simulink model "aa_IOT"  (R2024b)
settings: Solver=VariableStepAuto  StartTime=0.0  StopTime=0.05  RelTol=1e-3
undefined symbols (not defined in the file): Acid, Ion, Lead, Lithium, sigbuilder_block
libraries: spsBreakerLib x120, spsBatteryLib x82, spsSeriesRLCBranchLib x74, spsIdealSwitchLib x37, spsVoltageMeasurementLib x29, slpidlib x17, spsMosfetLib x17, spsPWMGeneratorDCDCLib x11, spsDiodeLib x10, spsIGBTLib x4, spsCurrentMeasurementLib x4, spsThreePhaseSeriesRLCLoadLib x2
(part 5 of 6)

== system aa_IOT/Grid/Wall charger Connection Box/DC-DC converter with battery controller/Battery controller ==
  Add1 : Sum  Inputs=+-
  Add2 : Sum  Inputs=+-
  Add3 : Sum  Inputs=+-
  Constant1 : Constant  Value=48
  Constant2 : Constant  Value=25.98
  Constant4 : Constant
  Current controller : slpidlib/PID Controller  Controller=PI  Form=Parallel  TimeDomain=Discrete-time  UseExternalTs=off  SampleTime=500e-6  IntegratorMethod=Forward Euler  FilterMethod=Forward Euler  ControllerParametersSource=internal  P=0.005  I=10  UseKiTs=off  D=0  UseExternalDerivativeSource=off  N=100  UseFilter=on  TunerSelectOption=Transfer Function Based (PID Tuner App)  InitialConditionSource=internal  InitialConditionForIntegrator=0.54  InitialConditionForFilter=0  DifferentiatorICPrevScaledInput=0  ExternalReset=none  TrackingMode=off  Kt=1  LimitOutput=on  SatLimitsSource=internal  UpperSaturationLimit=0.95  LowerSaturationLimit=0  LinearizeAsGain=on  AntiWindupMode=none  Kb=1  LimitIntegrator=off  UpperIntegratorSaturationLimit=inf  LowerIntegratorSaturationLimit=-inf  POutMin=[]  POutMax=[]  IOutMin=[]  IOutMax=[]  DOutMin=[]  DOutMax=[]  NOutMin=[]  NOutMax=[]  SumOutMin=[]  SumOutMax=[]  SaturationOutMin=[]  SaturationOutMax=[]  PParamMin=[]  PParamMax=[]  IParamMin=[]  IParamMax=[]  DParamMin=[]  DParamMax=[]  NParamMin=[]  NParamMax=[]  KbParamMin=[]  KbParamMax=[]  KtParamMin=[]  KtParamMax=[]  KbOutMin=[]  KbOutMax=[]  KtOutMin=[]  KtOutMax=[]  IntegratorOutMin=[]  IntegratorOutMax=[]  FilterOutMin=[]  FilterOutMax=[]  SumI1OutMin=[]  SumI1OutMax=[]  SumI2OutMin=[]  SumI2OutMax=[]  SumI3OutMin=[]  SumI3OutMax=[]  SumI4OutMin=[]  SumI4OutMax=[]  SumDOutMin=[]  SumDOutMax=[]  DifferentiatorOutMin=[]  DifferentiatorOutMax=[]  FilterDiffOutCoefMin=[]  FilterDiffOutCoefMax=[]  ReciprocalOutMin=[]  ReciprocalOutMax=[]  SumDenOutMin=[]  SumDenOutMax=[]  SumNumOutMin=[]  SumNumOutMax=[]  DivideOutMin=[]  DivideOutMax=[]  UdiffTsProdOutMin=[]  UdiffTsProdOutMax=[]  NTsProdOutMin=[]  NTsProdOutMax=[]  UintegralTsProdOutMin=[]  UintegralTsProdOutMax=[]  UngainTsProdOutMin=[]  UngainTsProdOutMax=[]  ClampingZeroOutDataTypeStr=Inherit: Inherit via back propagation  ClampingZeroOutMin=[]  ClampingZeroOutMax=[]  FilterDenConstantOutDataTypeStr=Inherit: Inherit via back propagation  FilterDenConstantOutMin=[]  FilterDenConstantOutMax=[]  PCopyOutDataTypeStr=Inherit: Inherit via back propagation  PCopyOutMin=[]  PCopyOutMax=[]  NCopyOutDataTypeStr=Inherit: Inherit via back propagation  NCopyOutMin=[]  NCopyOutMax=[]  IntegratorContinuousStateAttributes=''  IntegratorStateMustResolveToSignalObject=off  IntegratorRTWStateStorageClass=Auto  FilterContinuousStateAttributes=''  FilterStateMustResolveToSignalObject=off  FilterRTWStateStorageClass=Auto  ParallelPVariant=InternalParameters  IdealPVariant=Disabled  IVariant=InternalParameters  DVariant=Disabled  IntegratorVariant=Discrete  SatVariant=Enabled  AWVariant=Passthrough  PCopyVariant=Disabled  TRVariant=Disabled  FdbkBlocksVariant=Forward  IdealPFdbkVariant=Disabled  SatFdbkVariant=Disabled  DerivativeFilterVariant=Disabled  NVariant=Disabled  NCopyVariant=Disabled_SignalSpec  FilterICVariant=Disabled  IntegratorICVariant=InternalICs  ExternalResetVariant=Disabled  TRSumVariant=Passthrough  SumFdbkVariant=Disabled  SumVariant=Sum_PI  TsampFilterVariant=InternalTs  TsampNgainVariant=Passthrough  TsampIntegralVariant=Disabled_SignalSpec  ExternalSaturationOutDataTypeStr=Inherit: Same as second input  DerivativeSourceVariant=Disabled  PreIntVariant=InternalPreInt
  Display2 : Display
  Display3 : Display
  Display4 : Display
  Gain1 : Gain  Gain=-1
  NOT1 : Logic  Operator=NOT  IconShape=distinctive  AllPortsSameDT=off  OutDataTypeStr=boolean
  NOT3 : Logic  Operator=NOT  IconShape=distinctive  AllPortsSameDT=off  OutDataTypeStr=boolean
  PWM Generator (DC-DC)1 : spsPWMGeneratorDCDCLib/PWM Generator (DC-DC)  Fsw=10e3  Ts=5e-6
  Switch1 : Switch  Criteria=u2 > Threshold  SaturateOnIntegerOverflow=off  InputSameDT=off
  discharge controlled : slpidlib/PID Controller  Controller=PI  Form=Parallel  TimeDomain=Discrete-time  UseExternalTs=off  SampleTime=500e-6  IntegratorMethod=Forward Euler  FilterMethod=Forward Euler  ControllerParametersSource=internal  P=0.25  I=50  UseKiTs=off  D=0  UseExternalDerivativeSource=off  N=100  UseFilter=on  TunerSelectOption=Transfer Function Based (PID Tuner App)  InitialConditionSource=internal  InitialConditionForIntegrator=0  InitialConditionForFilter=0  DifferentiatorICPrevScaledInput=0  ExternalReset=none  TrackingMode=off  Kt=1  LimitOutput=on  SatLimitsSource=internal  UpperSaturationLimit=22  LowerSaturationLimit=0  LinearizeAsGain=on  AntiWindupMode=none  Kb=1  LimitIntegrator=off  UpperIntegratorSaturationLimit=inf  LowerIntegratorSaturationLimit=-inf  POutMin=[]  POutMax=[]  IOutMin=[]  IOutMax=[]  DOutMin=[]  DOutMax=[]  NOutMin=[]  NOutMax=[]  SumOutMin=[]  SumOutMax=[]  SaturationOutMin=[]  SaturationOutMax=[]  PParamMin=[]  PParamMax=[]  IParamMin=[]  IParamMax=[]  DParamMin=[]  DParamMax=[]  NParamMin=[]  NParamMax=[]  KbParamMin=[]  KbParamMax=[]  KtParamMin=[]  KtParamMax=[]  KbOutMin=[]  KbOutMax=[]  KtOutMin=[]  KtOutMax=[]  IntegratorOutMin=[]  IntegratorOutMax=[]  FilterOutMin=[]  FilterOutMax=[]  SumI1OutMin=[]  SumI1OutMax=[]  SumI2OutMin=[]  SumI2OutMax=[]  SumI3OutMin=[]  SumI3OutMax=[]  SumI4OutMin=[]  SumI4OutMax=[]  SumDOutMin=[]  SumDOutMax=[]  DifferentiatorOutMin=[]  DifferentiatorOutMax=[]  FilterDiffOutCoefMin=[]  FilterDiffOutCoefMax=[]  ReciprocalOutMin=[]  ReciprocalOutMax=[]  SumDenOutMin=[]  SumDenOutMax=[]  SumNumOutMin=[]  SumNumOutMax=[]  DivideOutMin=[]  DivideOutMax=[]  UdiffTsProdOutMin=[]  UdiffTsProdOutMax=[]  NTsProdOutMin=[]  NTsProdOutMax=[]  UintegralTsProdOutMin=[]  UintegralTsProdOutMax=[]  UngainTsProdOutMin=[]  UngainTsProdOutMax=[]  ClampingZeroOutDataTypeStr=Inherit: Inherit via back propagation  ClampingZeroOutMin=[]  ClampingZeroOutMax=[]  FilterDenConstantOutDataTypeStr=Inherit: Inherit via back propagation  FilterDenConstantOutMin=[]  FilterDenConstantOutMax=[]  PCopyOutDataTypeStr=Inherit: Inherit via back propagation  PCopyOutMin=[]  PCopyOutMax=[]  NCopyOutDataTypeStr=Inherit: Inherit via back propagation  NCopyOutMin=[]  NCopyOutMax=[]  IntegratorContinuousStateAttributes=''  IntegratorStateMustResolveToSignalObject=off  IntegratorRTWStateStorageClass=Auto  FilterContinuousStateAttributes=''  FilterStateMustResolveToSignalObject=off  FilterRTWStateStorageClass=Auto  ParallelPVariant=InternalParameters  IdealPVariant=Disabled  IVariant=InternalParameters  DVariant=Disabled  IntegratorVariant=Discrete  SatVariant=Enabled  AWVariant=Passthrough  PCopyVariant=Disabled  TRVariant=Disabled  FdbkBlocksVariant=Forward  IdealPFdbkVariant=Disabled  SatFdbkVariant=Disabled  DerivativeFilterVariant=Disabled  NVariant=Disabled  NCopyVariant=Disabled_SignalSpec  FilterICVariant=Disabled  IntegratorICVariant=InternalICs  ExternalResetVariant=Disabled  TRSumVariant=Passthrough  SumFdbkVariant=Disabled  SumVariant=Sum_PI  TsampFilterVariant=InternalTs  TsampNgainVariant=Passthrough  TsampIntegralVariant=Disabled_SignalSpec  ExternalSaturationOutDataTypeStr=Inherit: Same as second input  DerivativeSourceVariant=Disabled  PreIntVariant=InternalPreInt
  voltage controlled : slpidlib/PID Controller  Controller=PI  Form=Parallel  TimeDomain=Discrete-time  UseExternalTs=off  SampleTime=500e-6  IntegratorMethod=Forward Euler  FilterMethod=Forward Euler  ControllerParametersSource=internal  P=40  I=2000  UseKiTs=off  D=0  UseExternalDerivativeSource=off  N=100  UseFilter=on  TunerSelectOption=Transfer Function Based (PID Tuner App)  InitialConditionSource=internal  InitialConditionForIntegrator=0  InitialConditionForFilter=0  DifferentiatorICPrevScaledInput=0  ExternalReset=none  TrackingMode=off  Kt=1  LimitOutput=on  SatLimitsSource=internal  UpperSaturationLimit=22  LowerSaturationLimit=0  LinearizeAsGain=on  AntiWindupMode=none  Kb=1  LimitIntegrator=off  UpperIntegratorSaturationLimit=inf  LowerIntegratorSaturationLimit=-inf  POutMin=[]  POutMax=[]  IOutMin=[]  IOutMax=[]  DOutMin=[]  DOutMax=[]  NOutMin=[]  NOutMax=[]  SumOutMin=[]  SumOutMax=[]  SaturationOutMin=[]  SaturationOutMax=[]  PParamMin=[]  PParamMax=[]  IParamMin=[]  IParamMax=[]  DParamMin=[]  DParamMax=[]  NParamMin=[]  NParamMax=[]  KbParamMin=[]  KbParamMax=[]  KtParamMin=[]  KtParamMax=[]  KbOutMin=[]  KbOutMax=[]  KtOutMin=[]  KtOutMax=[]  IntegratorOutMin=[]  IntegratorOutMax=[]  FilterOutMin=[]  FilterOutMax=[]  SumI1OutMin=[]  SumI1OutMax=[]  SumI2OutMin=[]  SumI2OutMax=[]  SumI3OutMin=[]  SumI3OutMax=[]  SumI4OutMin=[]  SumI4OutMax=[]  SumDOutMin=[]  SumDOutMax=[]  DifferentiatorOutMin=[]  DifferentiatorOutMax=[]  FilterDiffOutCoefMin=[]  FilterDiffOutCoefMax=[]  ReciprocalOutMin=[]  ReciprocalOutMax=[]  SumDenOutMin=[]  SumDenOutMax=[]  SumNumOutMin=[]  SumNumOutMax=[]  DivideOutMin=[]  DivideOutMax=[]  UdiffTsProdOutMin=[]  UdiffTsProdOutMax=[]  NTsProdOutMin=[]  NTsProdOutMax=[]  UintegralTsProdOutMin=[]  UintegralTsProdOutMax=[]  UngainTsProdOutMin=[]  UngainTsProdOutMax=[]  ClampingZeroOutDataTypeStr=Inherit: Inherit via back propagation  ClampingZeroOutMin=[]  ClampingZeroOutMax=[]  FilterDenConstantOutDataTypeStr=Inherit: Inherit via back propagation  FilterDenConstantOutMin=[]  FilterDenConstantOutMax=[]  PCopyOutDataTypeStr=Inherit: Inherit via back propagation  PCopyOutMin=[]  PCopyOutMax=[]  NCopyOutDataTypeStr=Inherit: Inherit via back propagation  NCopyOutMin=[]  NCopyOutMax=[]  IntegratorContinuousStateAttributes=''  IntegratorStateMustResolveToSignalObject=off  IntegratorRTWStateStorageClass=Auto  FilterContinuousStateAttributes=''  FilterStateMustResolveToSignalObject=off  FilterRTWStateStorageClass=Auto  ParallelPVariant=InternalParameters  IdealPVariant=Disabled  IVariant=InternalParameters  DVariant=Disabled  IntegratorVariant=Discrete  SatVariant=Enabled  AWVariant=Passthrough  PCopyVariant=Disabled  TRVariant=Disabled  FdbkBlocksVariant=Forward  IdealPFdbkVariant=Disabled  SatFdbkVariant=Disabled  DerivativeFilterVariant=Disabled  NVariant=Disabled  NCopyVariant=Disabled_SignalSpec  FilterICVariant=Disabled  IntegratorICVariant=InternalICs  ExternalResetVariant=Disabled  TRSumVariant=Passthrough  SumFdbkVariant=Disabled  SumVariant=Sum_PI  TsampFilterVariant=InternalTs  TsampNgainVariant=Passthrough  TsampIntegralVariant=Disabled_SignalSpec  ExternalSaturationOutDataTypeStr=Inherit: Same as second input  DerivativeSourceVariant=Disabled  PreIntVariant=InternalPreInt
  tag scope: S_N=global, S_P=global
  wires:
  PWM Generator (DC-DC)1/1 -> NOT3/1, [S_P]
  voltage controlled/1 -> Gain1/1
  Constant2/1 -> Add3/1
  Add1/1 -> discharge controlled/1
  [Ib_ref_dis] -> Switch1/3
  Add2/1 -> Current controller/1
  [Ib_ref_charge] -> Switch1/1
  Add3/1 -> voltage controlled/1
  Switch1/1 -> Display4/1, [Ib_ref]
  [Ib_ref] -> Add2/2
  [Vb] -> Add3/2
  Gain1/1 -> Display3/1, [Ib_ref_charge]
  NOT3/1 -> [S_N]
  Constant1/1 -> Add1/1
  discharge controlled/1 -> Display2/1, [Ib_ref_dis]
  Current controller/1 -> PWM Generator (DC-DC)1/1
  [Ib] -> Add2/1
  [Vload] -> Add1/2
  [Control] -> NOT1/1
  NOT1/1 -> Switch1/2

== matlab function aa_IOT/Subsystem11/Swapping battery controller/MATLAB Function9 ==
  settings: updateMethod=DISCRETE
  data: SOC input; LoadOn output; ChargingOn output
function [LoadOn, ChargingOn] = chargeDischargeNode(SOC)
    % This function determines the charging and discharging states
    % based on the state of charge (SOC) of the battery.
    % Inputs:
    %   SOC - Current state of charge (0 to 100)
    % Outputs:
    %   LoadOn - Indicator if the load is on (1) or off (0)
    %   ChargingOn - Indicator if charging is active (1) or not (0)

    % Initialize persistent variables to retain state across function calls
    persistent LoadOnPersistent;
    persistent ChargingOnPersistent;

    if isempty(LoadOnPersistent)  % Initialize on first call
        LoadOnPersistent = 1;     % Load is initially on
        ChargingOnPersistent = 0;  % Charging is initially off
    end

    % Logic for charging and discharging based on SOC levels
    if SOC > 80
        LoadOnPersistent = 1;      % Turn load on if SOC is above 80%
        ChargingOnPersistent = 0;   % Turn charging off
    elseif SOC < 40
        LoadOnPersistent = 0;      % Turn load off if SOC is below 40%
        ChargingOnPersistent = 1;   % Start charging
    end

    % Assign output values from persistent variables
    LoadOn = LoadOnPersistent;
    ChargingOn = ChargingOnPersistent;
end

== matlab function aa_IOT/Subsystem11/Swapping battery controller/MATLAB Function10 ==
  settings: updateMethod=DISCRETE
  data: SOC input; LoadOn output; ChargingOn output
function [LoadOn, ChargingOn] = chargeDischargeNode(SOC)
    % This function determines the charging and discharging states
    % based on the state of charge (SOC) of the battery.
    % Inputs:
    %   SOC - Current state of charge (0 to 100)
    % Outputs:
    %   LoadOn - Indicator if the load is on (1) or off (0)
    %   ChargingOn - Indicator if charging is active (1) or not (0)

    % Initialize persistent variables to retain state across function calls
    persistent LoadOnPersistent;
    persistent ChargingOnPersistent;

    if isempty(LoadOnPersistent)  % Initialize on first call
        LoadOnPersistent = 1;     % Load is initially on
        ChargingOnPersistent = 0;  % Charging is initially off
    end

    % Logic for charging and discharging based on SOC levels
    if SOC > 80
        LoadOnPersistent = 1;      % Turn load on if SOC is above 80%
        ChargingOnPersistent = 0;   % Turn charging off
    elseif SOC < 40
        LoadOnPersistent = 0;      % Turn load off if SOC is below 40%
        ChargingOnPersistent = 1;   % Start charging
    end

    % Assign output values from persistent variables
    LoadOn = LoadOnPersistent;
    ChargingOn = ChargingOnPersistent;
end

== matlab function aa_IOT/Subsystem11/Swapping battery controller/MATLAB Function11 ==
  settings: updateMethod=DISCRETE
  data: SOC input; LoadOn output; ChargingOn output
function [LoadOn, ChargingOn] = chargeDischargeNode(SOC)
    % This function determines the charging and discharging states
    % based on the state of charge (SOC) of the battery.
    % Inputs:
    %   SOC - Current state of charge (0 to 100)
    % Outputs:
    %   LoadOn - Indicator if the load is on (1) or off (0)
    %   ChargingOn - Indicator if charging is active (1) or not (0)

    % Initialize persistent variables to retain state across function calls
    persistent LoadOnPersistent;
    persistent ChargingOnPersistent;

    if isempty(LoadOnPersistent)  % Initialize on first call
        LoadOnPersistent = 1;     % Load is initially on
        ChargingOnPersistent = 0;  % Charging is initially off
    end

    % Logic for charging and discharging based on SOC levels
    if SOC > 80
        LoadOnPersistent = 1;      % Turn load on if SOC is above 80%
        ChargingOnPersistent = 0;   % Turn charging off
    elseif SOC < 40
        LoadOnPersistent = 0;      % Turn load off if SOC is below 40%
        ChargingOnPersistent = 1;   % Start charging
    end

    % Assign output values from persistent variables
    LoadOn = LoadOnPersistent;
    ChargingOn = ChargingOnPersistent;
end

== matlab function aa_IOT/Subsystem11/Swapping battery controller/MATLAB Function12 ==
  settings: updateMethod=DISCRETE
  data: SOC input; LoadOn output; ChargingOn output
function [LoadOn, ChargingOn] = chargeDischargeNode(SOC)
    % This function determines the charging and discharging states
    % based on the state of charge (SOC) of the battery.
    % Inputs:
    %   SOC - Current state of charge (0 to 100)
    % Outputs:
    %   LoadOn - Indicator if the load is on (1) or off (0)
    %   ChargingOn - Indicator if charging is active (1) or not (0)

    % Initialize persistent variables to retain state across function calls
    persistent LoadOnPersistent;
    persistent ChargingOnPersistent;

    if isempty(LoadOnPersistent)  % Initialize on first call
        LoadOnPersistent = 1;     % Load is initially on
        ChargingOnPersistent = 0;  % Charging is initially off
    end

    % Logic for charging and discharging based on SOC levels
    if SOC > 80
        LoadOnPersistent = 1;      % Turn load on if SOC is above 80%
        ChargingOnPersistent = 0;   % Turn charging off
    elseif SOC < 40
        LoadOnPersistent = 0;      % Turn load off if SOC is below 40%
        ChargingOnPersistent = 1;   % Start charging
    end

    % Assign output values from persistent variables
    LoadOn = LoadOnPersistent;
    ChargingOn = ChargingOnPersistent;
end

== matlab function aa_IOT/Subsystem11/Swapping battery controller/MATLAB Function13 ==
  settings: updateMethod=DISCRETE
  data: SOC input; LoadOn output; ChargingOn output
function [LoadOn, ChargingOn] = chargeDischargeNode(SOC)
    % This function determines the charging and discharging states
    % based on the state of charge (SOC) of the battery.
    % Inputs:
    %   SOC - Current state of charge (0 to 100)
    % Outputs:
    %   LoadOn - Indicator if the load is on (1) or off (0)
    %   ChargingOn - Indicator if charging is active (1) or not (0)

    % Initialize persistent variables to retain state across function calls
    persistent LoadOnPersistent;
    persistent ChargingOnPersistent;

    if isempty(LoadOnPersistent)  % Initialize on first call
        LoadOnPersistent = 1;     % Load is initially on
        ChargingOnPersistent = 0;  % Charging is initially off
    end

    % Logic for charging and discharging based on SOC levels
    if SOC > 80
        LoadOnPersistent = 1;      % Turn load on if SOC is above 80%
        ChargingOnPersistent = 0;   % Turn charging off
    elseif SOC < 40
        LoadOnPersistent = 0;      % Turn load off if SOC is below 40%
        ChargingOnPersistent = 1;   % Start charging
    end

    % Assign output values from persistent variables
    LoadOn = LoadOnPersistent;
    ChargingOn = ChargingOnPersistent;
end

== matlab function aa_IOT/Subsystem11/Swapping battery controller/MATLAB Function14 ==
  settings: updateMethod=DISCRETE
  data: SOC input; LoadOn output; ChargingOn output
function [LoadOn, ChargingOn] = chargeDischargeNode(SOC)
    % This function determines the charging and discharging states
    % based on the state of charge (SOC) of the battery.
    % Inputs:
    %   SOC - Current state of charge (0 to 100)
    % Outputs:
    %   LoadOn - Indicator if the load is on (1) or off (0)
    %   ChargingOn - Indicator if charging is active (1) or not (0)

    % Initialize persistent variables to retain state across function calls
    persistent LoadOnPersistent;
    persistent ChargingOnPersistent;

    if isempty(LoadOnPersistent)  % Initialize on first call
        LoadOnPersistent = 1;     % Load is initially on
        ChargingOnPersistent = 0;  % Charging is initially off
    end

    % Logic for charging and discharging based on SOC levels
    if SOC > 80
        LoadOnPersistent = 1;      % Turn load on if SOC is above 80%
        ChargingOnPersistent = 0;   % Turn charging off
    elseif SOC < 40
        LoadOnPersistent = 0;      % Turn load off if SOC is below 40%
        ChargingOnPersistent = 1;   % Start charging
    end

    % Assign output values from persistent variables
    LoadOn = LoadOnPersistent;
    ChargingOn = ChargingOnPersistent;
end

== matlab function aa_IOT/Subsystem11/Swapping battery controller/MATLAB Function15 ==
  settings: updateMethod=DISCRETE
  data: SOC input; LoadOn output; ChargingOn output
function [LoadOn, ChargingOn] = chargeDischargeNode(SOC)
    % This function determines the charging and discharging states
    % based on the state of charge (SOC) of the battery.
    % Inputs:
    %   SOC - Current state of charge (0 to 100)
    % Outputs:
    %   LoadOn - Indicator if the load is on (1) or off (0)
    %   ChargingOn - Indicator if charging is active (1) or not (0)

    % Initialize persistent variables to retain state across function calls
    persistent LoadOnPersistent;
    persistent ChargingOnPersistent;

    if isempty(LoadOnPersistent)  % Initialize on first call
        LoadOnPersistent = 1;     % Load is initially on
        ChargingOnPersistent = 0;  % Charging is initially off
    end

    % Logic for charging and discharging based on SOC levels
    if SOC > 80
        LoadOnPersistent = 1;      % Turn load on if SOC is above 80%
        ChargingOnPersistent = 0;   % Turn charging off
    elseif SOC < 40
        LoadOnPersistent = 0;      % Turn load off if SOC is below 40%
        ChargingOnPersistent = 1;   % Start charging
    end

    % Assign output values from persistent variables
    LoadOn = LoadOnPersistent;
    ChargingOn = ChargingOnPersistent;
end

== matlab function aa_IOT/Subsystem11/Swapping battery controller/MATLAB Function16 ==
  settings: updateMethod=DISCRETE
  data: SOC input; LoadOn output; ChargingOn output
function [LoadOn, ChargingOn] = chargeDischargeNode(SOC)
    % This function determines the charging and discharging states
    % based on the state of charge (SOC) of the battery.
    % Inputs:
    %   SOC - Current state of charge (0 to 100)
    % Outputs:
    %   LoadOn - Indicator if the load is on (1) or off (0)
    %   ChargingOn - Indicator if charging is active (1) or not (0)

    % Initialize persistent variables to retain state across function calls
    persistent LoadOnPersistent;
    persistent ChargingOnPersistent;

    if isempty(LoadOnPersistent)  % Initialize on first call
        LoadOnPersistent = 1;     % Load is initially on
        ChargingOnPersistent = 0;  % Charging is initially off
    end

    % Logic for charging and discharging based on SOC levels
    if SOC > 80
        LoadOnPersistent = 1;      % Turn load on if SOC is above 80%
        ChargingOnPersistent = 0;   % Turn charging off
    elseif SOC < 40
        LoadOnPersistent = 0;      % Turn load off if SOC is below 40%
        ChargingOnPersistent = 1;   % Start charging
    end

    % Assign output values from persistent variables
    LoadOn = LoadOnPersistent;
    ChargingOn = ChargingOnPersistent;
end

== matlab function aa_IOT/Subsystem11/Swapping battery controller/MATLAB Function17 ==
  settings: updateMethod=DISCRETE
  data: SOC input; LoadOn output; ChargingOn output
function [LoadOn, ChargingOn] = chargeDischargeNode(SOC)
    % This function determines the charging and discharging states
    % based on the state of charge (SOC) of the battery.
    % Inputs:
    %   SOC - Current state of charge (0 to 100)
    % Outputs:
    %   LoadOn - Indicator if the load is on (1) or off (0)
    %   ChargingOn - Indicator if charging is active (1) or not (0)

    % Initialize persistent variables to retain state across function calls
    persistent LoadOnPersistent;
    persistent ChargingOnPersistent;

    if isempty(LoadOnPersistent)  % Initialize on first call
        LoadOnPersistent = 1;     % Load is initially on
        ChargingOnPersistent = 0;  % Charging is initially off
    end

    % Logic for charging and discharging based on SOC levels
    if SOC > 80
        LoadOnPersistent = 1;      % Turn load on if SOC is above 80%
        ChargingOnPersistent = 0;   % Turn charging off
    elseif SOC < 40
        LoadOnPersistent = 0;      % Turn load off if SOC is below 40%
        ChargingOnPersistent = 1;   % Start charging
    end

    % Assign output values from persistent variables
    LoadOn = LoadOnPersistent;
    ChargingOn = ChargingOnPersistent;
end

== matlab function aa_IOT/Subsystem11/Swapping battery controller/MATLAB Function18 ==
  settings: updateMethod=DISCRETE
  data: SOC input; LoadOn output; ChargingOn output
function [LoadOn, ChargingOn] = chargeDischargeNode(SOC)
    % This function determines the charging and discharging states
    % based on the state of charge (SOC) of the battery.
    % Inputs:
    %   SOC - Current state of charge (0 to 100)
    % Outputs:
    %   LoadOn - Indicator if the load is on (1) or off (0)
    %   ChargingOn - Indicator if charging is active (1) or not (0)

    % Initialize persistent variables to retain state across function calls
    persistent LoadOnPersistent;
    persistent ChargingOnPersistent;

    if isempty(LoadOnPersistent)  % Initialize on first call
        LoadOnPersistent = 1;     % Load is initially on
        ChargingOnPersistent = 0;  % Charging is initially off
    end

    % Logic for charging and discharging based on SOC levels
    if SOC > 80
        LoadOnPersistent = 1;      % Turn load on if SOC is above 80%
        ChargingOnPersistent = 0;   % Turn charging off
    elseif SOC < 40
        LoadOnPersistent = 0;      % Turn load off if SOC is below 40%
        ChargingOnPersistent = 1;   % Start charging
    end

    % Assign output values from persistent variables
    LoadOn = LoadOnPersistent;
    ChargingOn = ChargingOnPersistent;
end

== matlab function aa_IOT/Subsystem11/Swapping battery controller/MATLAB Function19 ==
  settings: updateMethod=DISCRETE
  data: SOC input; LoadOn output; ChargingOn output
function [LoadOn, ChargingOn] = chargeDischargeNode(SOC)
    % This function determines the charging and discharging states
    % based on the state of charge (SOC) of the battery.
    % Inputs:
    %   SOC - Current state of charge (0 to 100)
    % Outputs:
    %   LoadOn - Indicator if the load is on (1) or off (0)
    %   ChargingOn - Indicator if charging is active (1) or not (0)

    % Initialize persistent variables to retain state across function calls
    persistent LoadOnPersistent;
    persistent ChargingOnPersistent;

    if isempty(LoadOnPersistent)  % Initialize on first call
        LoadOnPersistent = 1;     % Load is initially on
        ChargingOnPersistent = 0;  % Charging is initially off
    end

    % Logic for charging and discharging based on SOC levels
    if SOC > 80
        LoadOnPersistent = 1;      % Turn load on if SOC is above 80%
        ChargingOnPersistent = 0;   % Turn charging off
    elseif SOC < 40
        LoadOnPersistent = 0;      % Turn load off if SOC is below 40%
        ChargingOnPersistent = 1;   % Start charging
    end

    % Assign output values from persistent variables
    LoadOn = LoadOnPersistent;
    ChargingOn = ChargingOnPersistent;
end

== matlab function aa_IOT/Subsystem11/Swapping battery controller/MATLAB Function20 ==
  settings: updateMethod=DISCRETE
  data: SOC input; LoadOn output; ChargingOn output
function [LoadOn, ChargingOn] = chargeDischargeNode(SOC)
    % This function determines the charging and discharging states
    % based on the state of charge (SOC) of the battery.
    % Inputs:
    %   SOC - Current state of charge (0 to 100)
    % Outputs:
    %   LoadOn - Indicator if the load is on (1) or off (0)
    %   ChargingOn - Indicator if charging is active (1) or not (0)

    % Initialize persistent variables to retain state across function calls
    persistent LoadOnPersistent;
    persistent ChargingOnPersistent;

    if isempty(LoadOnPersistent)  % Initialize on first call
        LoadOnPersistent = 1;     % Load is initially on
        ChargingOnPersistent = 0;  % Charging is initially off
    end

    % Logic for charging and discharging based on SOC levels
    if SOC > 80
        LoadOnPersistent = 1;      % Turn load on if SOC is above 80%
        ChargingOnPersistent = 0;   % Turn charging off
    elseif SOC < 40
        LoadOnPersistent = 0;      % Turn load off if SOC is below 40%
        ChargingOnPersistent = 1;   % Start charging
    end

    % Assign output values from persistent variables
    LoadOn = LoadOnPersistent;
    ChargingOn = ChargingOnPersistent;
end

== matlab function aa_IOT/Subsystem11/Swapping battery controller/MATLAB Function21 ==
  settings: updateMethod=DISCRETE
  data: SOC input; LoadOn output; ChargingOn output
function [LoadOn, ChargingOn] = chargeDischargeNode(SOC)
    % This function determines the charging and discharging states
    % based on the state of charge (SOC) of the battery.
    % Inputs:
    %   SOC - Current state of charge (0 to 100)
    % Outputs:
    %   LoadOn - Indicator if the load is on (1) or off (0)
    %   ChargingOn - Indicator if charging is active (1) or not (0)

    % Initialize persistent variables to retain state across function calls
    persistent LoadOnPersistent;
    persistent ChargingOnPersistent;

    if isempty(LoadOnPersistent)  % Initialize on first call
        LoadOnPersistent = 1;     % Load is initially on
        ChargingOnPersistent = 0;  % Charging is initially off
    end

    % Logic for charging and discharging based on SOC levels
    if SOC > 80
        LoadOnPersistent = 1;      % Turn load on if SOC is above 80%
        ChargingOnPersistent = 0;   % Turn charging off
    elseif SOC < 40
        LoadOnPersistent = 0;      % Turn load off if SOC is below 40%
        ChargingOnPersistent = 1;   % Start charging
    end

    % Assign output values from persistent variables
    LoadOn = LoadOnPersistent;
    ChargingOn = ChargingOnPersistent;
end

== matlab function aa_IOT/Subsystem11/Swapping battery controller/MATLAB Function22 ==
  settings: updateMethod=DISCRETE
  data: SOC input; LoadOn output; ChargingOn output
function [LoadOn, ChargingOn] = chargeDischargeNode(SOC)
    % This function determines the charging and discharging states
    % based on the state of charge (SOC) of the battery.
    % Inputs:
    %   SOC - Current state of charge (0 to 100)
    % Outputs:
    %   LoadOn - Indicator if the load is on (1) or off (0)
    %   ChargingOn - Indicator if charging is active (1) or not (0)

    % Initialize persistent variables to retain state across function calls
    persistent LoadOnPersistent;
    persistent ChargingOnPersistent;

    if isempty(LoadOnPersistent)  % Initialize on first call
        LoadOnPersistent = 1;     % Load is initially on
        ChargingOnPersistent = 0;  % Charging is initially off
    end

    % Logic for charging and discharging based on SOC levels
    if SOC > 80
        LoadOnPersistent = 1;      % Turn load on if SOC is above 80%
        ChargingOnPersistent = 0;   % Turn charging off
    elseif SOC < 40
        LoadOnPersistent = 0;      % Turn load off if SOC is below 40%
        ChargingOnPersistent = 1;   % Start charging
    end

    % Assign output values from persistent variables
    LoadOn = LoadOnPersistent;
    ChargingOn = ChargingOnPersistent;
end

== matlab function aa_IOT/Subsystem11/Swapping battery controller/MATLAB Function23 ==
  settings: updateMethod=DISCRETE
  data: SOC input; LoadOn output; ChargingOn output
function [LoadOn, ChargingOn] = chargeDischargeNode(SOC)
    % This function determines the charging and discharging states
    % based on the state of charge (SOC) of the battery.
    % Inputs:
    %   SOC - Current state of charge (0 to 100)
    % Outputs:
    %   LoadOn - Indicator if the load is on (1) or off (0)
    %   ChargingOn - Indicator if charging is active (1) or not (0)

    % Initialize persistent variables to retain state across function calls
    persistent LoadOnPersistent;
    persistent ChargingOnPersistent;

    if isempty(LoadOnPersistent)  % Initialize on first call
        LoadOnPersistent = 1;     % Load is initially on
        ChargingOnPersistent = 0;  % Charging is initially off
    end

    % Logic for charging and discharging based on SOC levels
    if SOC > 80
        LoadOnPersistent = 1;      % Turn load on if SOC is above 80%
        ChargingOnPersistent = 0;   % Turn charging off
    elseif SOC < 40
        LoadOnPersistent = 0;      % Turn load off if SOC is below 40%
        ChargingOnPersistent = 1;   % Start charging
    end

    % Assign output values from persistent variables
    LoadOn = LoadOnPersistent;
    ChargingOn = ChargingOnPersistent;
end

== matlab function aa_IOT/Solar/MPPT/Embedded MATLAB Function1 ==
  settings: updateMethod=DISCRETE
  data: V input; I input; T input; D output
function D   = PO(V,I,T)
persistent P2  P1  dP d dd n;
if isempty(V)
    V=370;
end
if isempty(I)
    I=0;
end
if isempty(P2)
    P2=0;
end
if isempty(P1)
    P1=0;
end
if isempty(dP)
    dP=0;
end
if isempty(d)
    d=1;
end
if isempty(dd)
    dd=0;
end
if isempty(n)
    n=1;
end
%%%%%%%%%%%%%%%%%%%%%
    if  (T > n*0.02)   %chu ki lay mau 0.02s
    n = n + 1;
    P1=P2;
    P2=V*I;
    dP=P2-P1;
    if (dd==0)
        if dP>1
            dd=0.01;
            d=d+dd;
        else
            if dP<-1
                dd=-0.01;
                d=d+dd;
            else
                dd=0;
            end
        end
    else
        if ((dP<1)&&(dP>-1))
        dd=0;
        d=d+dd;
        else
            if ((dP/dd)>0)
                dd=0.01;
                d=d+dd;
            else
                dd=-0.01;
                d=d+dd;
            end
        end
    end    
    end
D=d/(d+1);
if D<0.4
    D=0.4;
    d=D/(1-D);
else
    if D>0.9
        D=0.9;
        d=D/(1-D);
    else
    end
end
end

== matlab function aa_IOT/Subsystem11/Swapping battery controller/MATLAB Function24 ==
  settings: updateMethod=DISCRETE
  data: SOC input; LoadOn output; ChargingOn output
function [LoadOn, ChargingOn] = chargeDischargeNode(SOC)
    % This function determines the charging and discharging states
    % based on the state of charge (SOC) of the battery.
    % Inputs:
    %   SOC - Current state of charge (0 to 100)
    % Outputs:
    %   LoadOn - Indicator if the load is on (1) or off (0)
    %   ChargingOn - Indicator if charging is active (1) or not (0)

    % Initialize persistent variables to retain state across function calls
    persistent LoadOnPersistent;
    persistent ChargingOnPersistent;

    if isempty(LoadOnPersistent)  % Initialize on first call
        LoadOnPersistent = 1;     % Load is initially on
        ChargingOnPersistent = 0;  % Charging is initially off
    end

    % Logic for charging and discharging based on SOC levels
    if SOC > 80
        LoadOnPersistent = 1;      % Turn load on if SOC is above 80%
        ChargingOnPersistent = 0;   % Turn charging off
    elseif SOC < 40
        LoadOnPersistent = 0;      % Turn load off if SOC is below 40%
        ChargingOnPersistent = 1;   % Start charging
    end

    % Assign output values from persistent variables
    LoadOn = LoadOnPersistent;
    ChargingOn = ChargingOnPersistent;
end

== matlab function aa_IOT/Subsystem11/Swapping battery controller/MATLAB Function25 ==
  settings: updateMethod=DISCRETE
  data: SOC input; LoadOn output; ChargingOn output
function [LoadOn, ChargingOn] = chargeDischargeNode(SOC)
    % This function determines the charging and discharging states
    % based on the state of charge (SOC) of the battery.
    % Inputs:
    %   SOC - Current state of charge (0 to 100)
    % Outputs:
    %   LoadOn - Indicator if the load is on (1) or off (0)
    %   ChargingOn - Indicator if charging is active (1) or not (0)

    % Initialize persistent variables to retain state across function calls
    persistent LoadOnPersistent;
    persistent ChargingOnPersistent;

    if isempty(LoadOnPersistent)  % Initialize on first call
        LoadOnPersistent = 1;     % Load is initially on
        ChargingOnPersistent = 0;  % Charging is initially off
    end

    % Logic for charging and discharging based on SOC levels
    if SOC > 80
        LoadOnPersistent = 1;      % Turn load on if SOC is above 80%
        ChargingOnPersistent = 0;   % Turn charging off
    elseif SOC < 40
        LoadOnPersistent = 0;      % Turn load off if SOC is below 40%
        ChargingOnPersistent = 1;   % Start charging
    end

    % Assign output values from persistent variables
    LoadOn = LoadOnPersistent;
    ChargingOn = ChargingOnPersistent;
end

== matlab function aa_IOT/Subsystem11/Swapping battery controller/MATLAB Function26 ==
  settings: updateMethod=DISCRETE
  data: SOC input; LoadOn output; ChargingOn output
function [LoadOn, ChargingOn] = chargeDischargeNode(SOC)
    % This function determines the charging and discharging states
    % based on the state of charge (SOC) of the battery.
    % Inputs:
    %   SOC - Current state of charge (0 to 100)
    % Outputs:
    %   LoadOn - Indicator if the load is on (1) or off (0)
    %   ChargingOn - Indicator if charging is active (1) or not (0)

    % Initialize persistent variables to retain state across function calls
    persistent LoadOnPersistent;
    persistent ChargingOnPersistent;

    if isempty(LoadOnPersistent)  % Initialize on first call
        LoadOnPersistent = 1;     % Load is initially on
        ChargingOnPersistent = 0;  % Charging is initially off
    end

    % Logic for charging and discharging based on SOC levels
    if SOC > 80
        LoadOnPersistent = 1;      % Turn load on if SOC is above 80%
        ChargingOnPersistent = 0;   % Turn charging off
    elseif SOC < 40
        LoadOnPersistent = 0;      % Turn load off if SOC is below 40%
        ChargingOnPersistent = 1;   % Start charging
    end

    % Assign output values from persistent variables
    LoadOn = LoadOnPersistent;
    ChargingOn = ChargingOnPersistent;
end

== matlab function aa_IOT/Subsystem11/Swapping battery controller/MATLAB Function27 ==
  settings: updateMethod=DISCRETE
  data: SOC input; LoadOn output; ChargingOn output
function [LoadOn, ChargingOn] = chargeDischargeNode(SOC)
    % This function determines the charging and discharging states
    % based on the state of charge (SOC) of the battery.
    % Inputs:
    %   SOC - Current state of charge (0 to 100)
    % Outputs:
    %   LoadOn - Indicator if the load is on (1) or off (0)
    %   ChargingOn - Indicator if charging is active (1) or not (0)

    % Initialize persistent variables to retain state across function calls
    persistent LoadOnPersistent;
    persistent ChargingOnPersistent;

    if isempty(LoadOnPersistent)  % Initialize on first call
        LoadOnPersistent = 1;     % Load is initially on
        ChargingOnPersistent = 0;  % Charging is initially off
    end

    % Logic for charging and discharging based on SOC levels
    if SOC > 80
        LoadOnPersistent = 1;      % Turn load on if SOC is above 80%
        ChargingOnPersistent = 0;   % Turn charging off
    elseif SOC < 40
        LoadOnPersistent = 0;      % Turn load off if SOC is below 40%
        ChargingOnPersistent = 1;   % Start charging
    end

    % Assign output values from persistent variables
    LoadOn = LoadOnPersistent;
    ChargingOn = ChargingOnPersistent;
end

== matlab function aa_IOT/Subsystem11/Swapping battery controller/MATLAB Function28 ==
  settings: updateMethod=DISCRETE
  data: SOC input; LoadOn output; ChargingOn output
function [LoadOn, ChargingOn] = chargeDischargeNode(SOC)
    % This function determines the charging and discharging states
    % based on the state of charge (SOC) of the battery.
    % Inputs:
    %   SOC - Current state of charge (0 to 100)
    % Outputs:
    %   LoadOn - Indicator if the load is on (1) or off (0)
    %   ChargingOn - Indicator if charging is active (1) or not (0)

    % Initialize persistent variables to retain state across function calls
    persistent LoadOnPersistent;
    persistent ChargingOnPersistent;

    if isempty(LoadOnPersistent)  % Initialize on first call
        LoadOnPersistent = 1;     % Load is initially on
        ChargingOnPersistent = 0;  % Charging is initially off
    end

    % Logic for charging and discharging based on SOC levels
    if SOC > 80
        LoadOnPersistent = 1;      % Turn load on if SOC is above 80%
        ChargingOnPersistent = 0;   % Turn charging off
    elseif SOC < 40
        LoadOnPersistent = 0;      % Turn load off if SOC is below 40%
        ChargingOnPersistent = 1;   % Start charging
    end

    % Assign output values from persistent variables
    LoadOn = LoadOnPersistent;
    ChargingOn = ChargingOnPersistent;
end

== matlab function aa_IOT/Subsystem11/Swapping battery controller/MATLAB Function29 ==
  settings: updateMethod=DISCRETE
  data: SOC input; LoadOn output; ChargingOn output
function [LoadOn, ChargingOn] = chargeDischargeNode(SOC)
    % This function determines the charging and discharging states
    % based on the state of charge (SOC) of the battery.
    % Inputs:
    %   SOC - Current state of charge (0 to 100)
    % Outputs:
    %   LoadOn - Indicator if the load is on (1) or off (0)
    %   ChargingOn - Indicator if charging is active (1) or not (0)

    % Initialize persistent variables to retain state across function calls
    persistent LoadOnPersistent;
    persistent ChargingOnPersistent;

    if isempty(LoadOnPersistent)  % Initialize on first call
        LoadOnPersistent = 1;     % Load is initially on
        ChargingOnPersistent = 0;  % Charging is initially off
    end

    % Logic for charging and discharging based on SOC levels
    if SOC > 80
        LoadOnPersistent = 1;      % Turn load on if SOC is above 80%
        ChargingOnPersistent = 0;   % Turn charging off
    elseif SOC < 40
        LoadOnPersistent = 0;      % Turn load off if SOC is below 40%
        ChargingOnPersistent = 1;   % Start charging
    end

    % Assign output values from persistent variables
    LoadOn = LoadOnPersistent;
    ChargingOn = ChargingOnPersistent;
end

== matlab function aa_IOT/Subsystem4/Subsystem/MATLAB Function ==
  data: u1 input; s1 output; u2 input; u3 input; s2 output; s3 output
function [s1, s2, s3] = fcn(u1, u2, u3)
    u1 = int32(u1);
    u2 = int32(u2);
    u3 = int32(u3);

    if (u1 > u2 || u1 > u3)
        s1 = 1;
    else
        s1 = 0;
    end

    if (u2 > u1 || u2 > u3)
        s2 = 1;
    else
        s2 = 0;
    end

    if (u3 > u1 || u3 > u2)
        s3 = 1;
    else
        s3 = 0;
    end
end

== matlab function aa_IOT/Subsystem5/Subsystem/MATLAB Function ==
  data: u1 input; s1 output; u2 input; u3 input; s2 output; s3 output
function [s1, s2, s3] = fcn(u1, u2, u3)
    u1 = int32(u1);
    u2 = int32(u2);
    u3 = int32(u3);

    if (u1 > u2 || u1 > u3)
        s1 = 1;
    else
        s1 = 0;
    end

    if (u2 > u1 || u2 > u3)
        s2 = 1;
    else
        s2 = 0;
    end

    if (u3 > u1 || u3 > u2)
        s3 = 1;
    else
        s3 = 0;
    end
end

== matlab function aa_IOT/Subsystem6/Subsystem/MATLAB Function ==
  data: u1 input; s1 output; u2 input; u3 input; s2 output; s3 output
function [s1, s2, s3] = fcn(u1, u2, u3)
    u1 = int32(u1);
    u2 = int32(u2);
    u3 = int32(u3);

    if (u1 > u2 || u1 > u3)
        s1 = 1;
    else
        s1 = 0;
    end

    if (u2 > u1 || u2 > u3)
        s2 = 1;
    else
        s2 = 0;
    end

    if (u3 > u1 || u3 > u2)
        s3 = 1;
    else
        s3 = 0;
    end
end

== matlab function aa_IOT/Subsystem7/Subsystem/MATLAB Function ==
  data: u1 input; s1 output; u2 input; u3 input; s2 output; s3 output
function [s1, s2, s3] = fcn(u1, u2, u3)
    u1 = int32(u1);
    u2 = int32(u2);
    u3 = int32(u3);

    if (u1 > u2 || u1 > u3)
        s1 = 1;
    else
        s1 = 0;
    end

    if (u2 > u1 || u2 > u3)
        s2 = 1;
    else
        s2 = 0;
    end

    if (u3 > u1 || u3 > u2)
        s3 = 1;
    else
        s3 = 0;
    end
end

== matlab function aa_IOT/Subsystem11/Swapping battery controller/MATLAB Function ==
  settings: updateMethod=DISCRETE
  data: SOC input; LoadOn output; ChargingOn output
function [LoadOn, ChargingOn] = chargeDischargeNode(SOC)
    % This function determines the charging and discharging states
    % based on the state of charge (SOC) of the battery.
    % Inputs:
    %   SOC - Current state of charge (0 to 100)
    % Outputs:
    %   LoadOn - Indicator if the load is on (1) or off (0)
    %   ChargingOn - Indicator if charging is active (1) or not (0)

    % Initialize persistent variables to retain state across function calls
    persistent LoadOnPersistent;
    persistent ChargingOnPersistent;

    if isempty(LoadOnPersistent)  % Initialize on first call
        LoadOnPersistent = 1;     % Load is initially on
        ChargingOnPersistent = 0;  % Charging is initially off
    end

    % Logic for charging and discharging based on SOC levels
    if SOC > 80
        LoadOnPersistent = 1;      % Turn load on if SOC is above 80%
        ChargingOnPersistent = 0;   % Turn charging off
    elseif SOC < 40
        LoadOnPersistent = 0;      % Turn load off if SOC is below 40%
        ChargingOnPersistent = 1;   % Start charging
    end

    % Assign output values from persistent variables
    LoadOn = LoadOnPersistent;
    ChargingOn = ChargingOnPersistent;
end

== matlab function aa_IOT/Grid/Wall charger Connection Box/DC-AC // AC-DC Converter/Controller/MATLAB Function ==
  data: x input; a output; b output; ma input; shift input; c output
function [a,b,c] = ref_generation(x,ma,shift)

shift_k=shift*pi/180;
a=(ma*(sin((x)+shift_k)));
b=(ma*(sin((x)+shift_k-(2*pi/3))));
c=(ma*(sin((x)+shift_k+(2*pi/3))));

== matlab function aa_IOT/Subsystem11/Swapping battery controller/MATLAB Function1 ==
  settings: updateMethod=DISCRETE
  data: SOC input; LoadOn output; ChargingOn output
function [LoadOn, ChargingOn] = chargeDischargeNode(SOC)
    % This function determines the charging and discharging states
    % based on the state of charge (SOC) of the battery.
    % Inputs:
    %   SOC - Current state of charge (0 to 100)
    % Outputs:
    %   LoadOn - Indicator if the load is on (1) or off (0)
    %   ChargingOn - Indicator if charging is active (1) or not (0)

    % Initialize persistent variables to retain state across function calls
    persistent LoadOnPersistent;
    persistent ChargingOnPersistent;

    if isempty(LoadOnPersistent)  % Initialize on first call
        LoadOnPersistent = 1;     % Load is initially on
        ChargingOnPersistent = 0;  % Charging is initially off
    end

    % Logic for charging and discharging based on SOC levels
    if SOC > 80
        LoadOnPersistent = 1;      % Turn load on if SOC is above 80%
        ChargingOnPersistent = 0;   % Turn charging off
    elseif SOC < 40
        LoadOnPersistent = 0;      % Turn load off if SOC is below 40%
        ChargingOnPersistent = 1;   % Start charging
    end

    % Assign output values from persistent variables
    LoadOn = LoadOnPersistent;
    ChargingOn = ChargingOnPersistent;
end

== matlab function aa_IOT/Subsystem11/Swapping battery controller/MATLAB Function2 ==
  settings: updateMethod=DISCRETE
  data: SOC input; LoadOn output; ChargingOn output
function [LoadOn, ChargingOn] = chargeDischargeNode(SOC)
    % This function determines the charging and discharging states
    % based on the state of charge (SOC) of the battery.
    % Inputs:
    %   SOC - Current state of charge (0 to 100)
    % Outputs:
    %   LoadOn - Indicator if the load is on (1) or off (0)
    %   ChargingOn - Indicator if charging is active (1) or not (0)

    % Initialize persistent variables to retain state across function calls
    persistent LoadOnPersistent;
    persistent ChargingOnPersistent;

    if isempty(LoadOnPersistent)  % Initialize on first call
        LoadOnPersistent = 1;     % Load is initially on
        ChargingOnPersistent = 0;  % Charging is initially off
    end

    % Logic for charging and discharging based on SOC levels
    if SOC > 80
        LoadOnPersistent = 1;      % Turn load on if SOC is above 80%
        ChargingOnPersistent = 0;   % Turn charging off
    elseif SOC < 40
        LoadOnPersistent = 0;      % Turn load off if SOC is below 40%
        ChargingOnPersistent = 1;   % Start charging
    end

    % Assign output values from persistent variables
    LoadOn = LoadOnPersistent;
    ChargingOn = ChargingOnPersistent;
end

== matlab function aa_IOT/Subsystem11/Swapping battery controller/MATLAB Function3 ==
  settings: updateMethod=DISCRETE
  data: SOC input; LoadOn output; ChargingOn output
function [LoadOn, ChargingOn] = chargeDischargeNode(SOC)
    % This function determines the charging and discharging states
    % based on the state of charge (SOC) of the battery.
    % Inputs:
    %   SOC - Current state of charge (0 to 100)
    % Outputs:
    %   LoadOn - Indicator if the load is on (1) or off (0)
    %   ChargingOn - Indicator if charging is active (1) or not (0)

    % Initialize persistent variables to retain state across function calls
    persistent LoadOnPersistent;
    persistent ChargingOnPersistent;

    if isempty(LoadOnPersistent)  % Initialize on first call
        LoadOnPersistent = 1;     % Load is initially on
        ChargingOnPersistent = 0;  % Charging is initially off
    end

    % Logic for charging and discharging based on SOC levels
    if SOC > 80
        LoadOnPersistent = 1;      % Turn load on if SOC is above 80%
        ChargingOnPersistent = 0;   % Turn charging off
    elseif SOC < 40
        LoadOnPersistent = 0;      % Turn load off if SOC is below 40%
        ChargingOnPersistent = 1;   % Start charging
    end

    % Assign output values from persistent variables
    LoadOn = LoadOnPersistent;
    ChargingOn = ChargingOnPersistent;
end
